simulink model "ADRC5linESO"  (R2016a)
settings: Solver=VariableStepAuto  StartTime=0.0  StopTime=5.0  RelTol=1e-3
undefined symbols (not defined in the file or in its folder): Ts, wn, zn
settings Model: Creator=User  LastModifiedBy=User

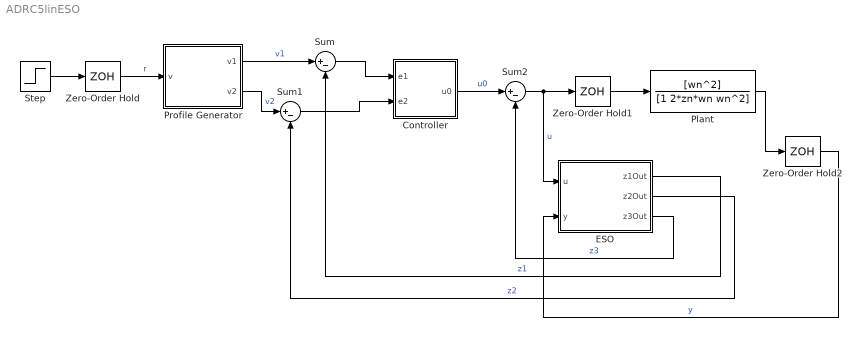
== system ADRC5linESO ==
  Controller : Subsystem
  ESO : Subsystem
  Plant : TransferFcn  Numerator=[wn^2]  Denominator=[1 2*zn*wn wn^2]
  Profile Generator : Subsystem
  Step : Step  SampleTime=0
  Sum : Sum  Inputs=|+-
  Sum1 : Sum  Inputs=|+-
  Sum2 : Sum  Inputs=|+-
  Zero-Order Hold : ZeroOrderHold  SampleTime=Ts
  Zero-Order Hold1 : ZeroOrderHold  SampleTime=Ts
  Zero-Order Hold2 : ZeroOrderHold  SampleTime=Ts
  wires:
  Step/1 -> Zero-Order Hold/1
  Zero-Order Hold/1 -> Profile Generator/1(v)  "r"
  Profile Generator/1(v1) -> Sum/1  "v1"
  Profile Generator/2(v2) -> Sum1/1  "v2"
  ESO/2(z2Out) -> Sum1/2  "z2"
  ESO/1(z1Out) -> Sum/2  "z1"
  ESO/3(z3Out) -> Sum2/2  "z3"
  Sum2/1 -> Zero-Order Hold1/1, ESO/1(u)  "u"
  Zero-Order Hold1/1 -> Plant/1
  Plant/1 -> Zero-Order Hold2/1
  Zero-Order Hold2/1 -> ESO/2(y)  "y"
  Sum/1 -> Controller/1(e1)
  Sum1/1 -> Controller/2(e2)
  Controller/1(u0) -> Sum2/1  "u0"

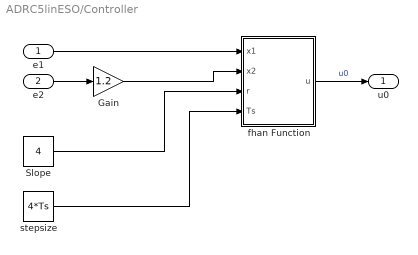
== system ADRC5linESO/Controller ==
  e1 : Inport
  e2 : Inport  Port=2
  Gain : Gain  Gain=1.2
  Slope : Constant  Value=4
  fhan Function : MATLAB Function  TreatAsAtomicUnit=on
  stepsize : Constant  Value=4*Ts
  u0 : Outport
  wires:
  e2/1 -> Gain/1
  stepsize/1 -> fhan Function/4(Ts)
  Slope/1 -> fhan Function/3(r)
  e1/1 -> fhan Function/1(x1)
  fhan Function/1(u) -> u0/1  "u0"
  Gain/1 -> fhan Function/2(x2)

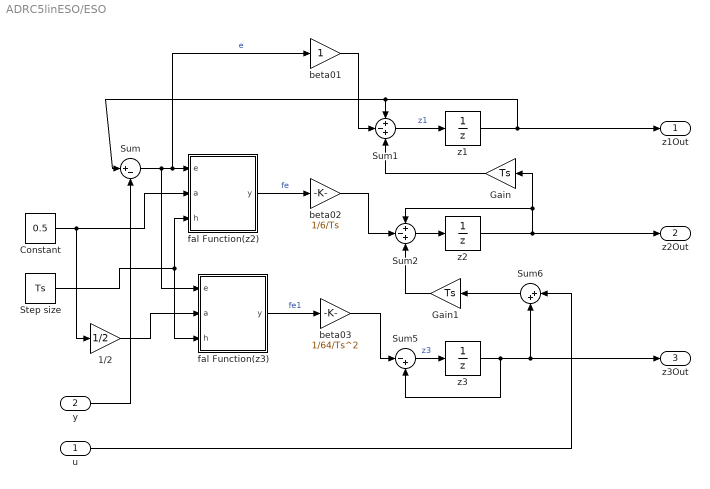
== system ADRC5linESO/ESO ==
  u : Inport
  y : Inport  Port=2
  1/2 : Gain  Gain=1/2
  Constant : Constant  Value=0.5
  Gain : Gain  Gain=Ts
  Gain1 : Gain  Gain=Ts
  Step size : Constant  Value=Ts
  Sum : Sum  Inputs=|+-
  Sum1 : Sum  Inputs=+-+
  Sum2 : Sum  Inputs=+-+
  Sum5 : Sum  Inputs=|-+
  Sum6 : Sum  Inputs=|++
  beta01 : Gain
  beta02 : Gain  Gain=1/6/Ts
  beta03 : Gain  Gain=1/64/Ts^2
  fal Function(z2) : MATLAB Function  TreatAsAtomicUnit=on
  fal Function(z3) : MATLAB Function  TreatAsAtomicUnit=on
  z1 : UnitDelay  SampleTime=Ts
  z2 : UnitDelay  SampleTime=Ts
  z3 : UnitDelay  SampleTime=Ts
  z1Out : Outport
  z2Out : Outport  Port=2
  z3Out : Outport  Port=3
  wires:
  z2/1 -> Sum2/1, Gain/1, z2Out/1
  z1/1 -> Sum1/1, Sum/1, z1Out/1
  z3/1 -> Sum6/2, z3Out/1, Sum5/2
  Constant/1 -> 1/2/1, fal Function(z2)/2(a)
  Sum/1 -> fal Function(z3)/1(e), beta01/1, fal Function(z2)/1(e)  "e"
  Step size/1 -> fal Function(z3)/3(h), fal Function(z2)/3(h)
  1/2/1 -> fal Function(z3)/2(a)
  fal Function(z2)/1(y) -> beta02/1  "fe"
  fal Function(z3)/1(y) -> beta03/1  "fe1"
  u/1 -> Sum6/1
  beta01/1 -> Sum1/2
  y/1 -> Sum/2
  Sum1/1 -> z1/1  "z1"
  Sum2/1 -> z2/1
  Sum5/1 -> z3/1  "z3"
  beta03/1 -> Sum5/1
  Sum6/1 -> Gain1/1
  Gain1/1 -> Sum2/3
  beta02/1 -> Sum2/2
  Gain/1 -> Sum1/3

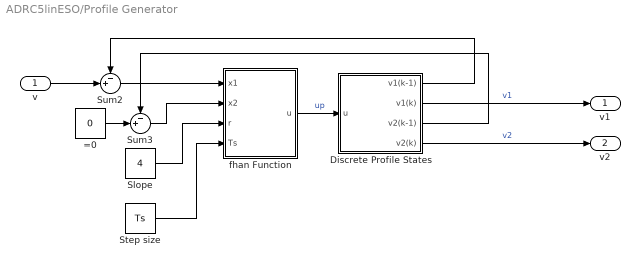
== system ADRC5linESO/Profile Generator ==
  v : Inport
  =0 : Constant  Value=0
  Discrete Profile States : Subsystem
  Slope : Constant  Value=4
  Step size : Constant  Value=Ts
  Sum2 : Sum  Inputs=-+|
  Sum3 : Sum  Inputs=-+|
  fhan Function : MATLAB Function  TreatAsAtomicUnit=on
  v1 : Outport
  v2 : Outport  Port=2
  wires:
  Sum2/1 -> fhan Function/1(x1)
  Sum3/1 -> fhan Function/2(x2)
  Step size/1 -> fhan Function/4(Ts)
  Discrete Profile States/3(v2(k-1)) -> Sum3/1
  Discrete Profile States/4(v2(k)) -> v2/1  "v2"
  Discrete Profile States/2(v1(k)) -> v1/1  "v1"
  fhan Function/1(u) -> Discrete Profile States/1(u)  "up"
  Discrete Profile States/1(v1(k-1)) -> Sum2/1
  v/1 -> Sum2/2
  =0/1 -> Sum3/2
  Slope/1 -> fhan Function/3(r)

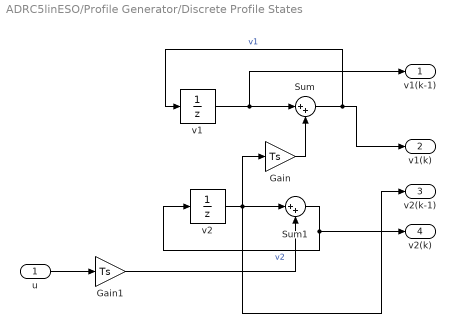
== system ADRC5linESO/Profile Generator/Discrete Profile States ==
  u : Inport
  Gain : Gain  Gain=Ts
  Gain1 : Gain  Gain=Ts
  Sum : Sum  Inputs=|++
  Sum1 : Sum  Inputs=|++
  v1 : UnitDelay  SampleTime=Ts
  v2 : UnitDelay  SampleTime=Ts
  v1(k-1) : Outport
  v1(k) : Outport  Port=2
  v2(k-1) : Outport  Port=3
  v2(k) : Outport  Port=4
  wires:
  Sum/1 -> v1(k)/1, v1/1  "v1"
  Gain/1 -> Sum/2
  Sum1/1 -> v2(k)/1, v2/1  "v2"
  u/1 -> Gain1/1
  v2/1 -> Gain/1, v2(k-1)/1, Sum1/1
  v1/1 -> v1(k-1)/1, Sum/1
  Gain1/1 -> Sum1/2

== matlab function ADRC5linESO/ESO/fal Function(z2) ==
  data: e input; y output; a input; h input
function y = fal(e,a,h)
%#codegen

ae = abs(e);
if (ae <= h)
    a1 = 1 - a;
    y = e/(h^a1);
else
    y = (abs(e)^a)*sign(e);
end
y=e;        % Override for linear function (comment out for non-linear)

== matlab function ADRC5linESO/Profile Generator/fhan Function ==
  data: x1 input; x2 input; u output; r input; Ts input
function u = tod(x1,x2,r,Ts)
%#codegen
d = Ts*r;
d0= Ts*d;
y = x1+Ts*x2;
ya= abs(y);
a0= sqrt(d^2 + 8*r*ya);
if (ya > d0),
    a = x2 + (a0-d)/2*sign(y);
else
    a = x2 + y/Ts;
end
aa = abs(a);
if (aa > d),
    fst = r*sign(a);
else
    fst = r*a/d;
end
   
u = fst;

== matlab function ADRC5linESO/ESO/fal Function(z3) ==
  data: e input; y output; a input; h input
function y = fal(e,a,h)
%#codegen

ae = abs(e);
if (ae <= h)
    a1 = 1 - a;
    y = e/(h^a1);
else
    y = (abs(e)^a)*sign(e);
end
y = e;        % Override for linear function (comment out for non-linear)

== matlab function ADRC5linESO/Controller/fhan Function ==
  data: x1 input; x2 input; u output; r input; Ts input
function u = tod(x1,x2,r,Ts)
%#codegen
d = Ts*r;
d0= Ts*d;
y = x1+Ts*x2;
ya=abs(y);
a0= sqrt(d^2 + 8*r*ya);
if (ya > d0),
    a = x2 + (a0-d)/2*sign(y);
else
    a = x2 + y/Ts;
end
aa = abs(a);
if (aa > d),
    fst = r*sign(a);
else
    fst = r*a/d;
end
   
u = fst;
